simulink model "state_machine_with_obstacle"  (R2016a)
settings: Solver=FixedStepDiscrete  StartTime=0.0  StopTime=100  FixedStep=0.01  MaxStep=0.01  RelTol=1e-3
undefined symbols (not defined in the file): track_3
libraries: lflib x13
settings Model: Creator=The MathWorks, Inc.  LastModifiedBy=bures
settings SolverCC: ZeroCrossAlgorithm=Adaptive
settings DataIOCC: LimitDataPoints=on
settings DebuggingCC: AllowSymbolicDim=off
settings ModelReferenceCC: PropagateSignalLabelsOutOfModel=off
settings GRTTargetCC: GeneratePreprocessorConditionals=Use local settings

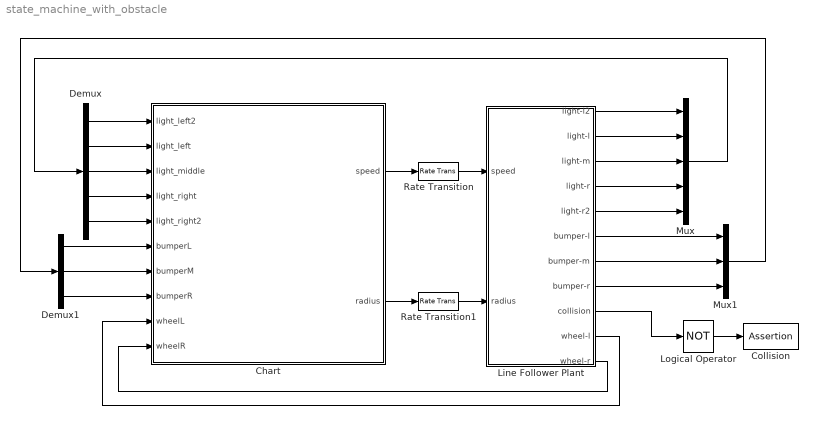
== system state_machine_with_obstacle ==
  Chart : Stateflow chart  TreatAsAtomicUnit=on
  Collision : Assertion
  Demux : Demux  Outputs=5
  Demux1 : Demux  Outputs=3
  Line Follower Plant : Subsystem  mask{initX=506, initY=1050, initAngle=3/2*pi, trackCData=track_3, trackSamplesPerM=1000}
      mask prompts: initX "X (in mm)"; initY "Y (in mm)"; initAngle "Angle (in rad)"; trackCData "Track map"; trackSamplesPerM "Track map samples/m"
  Logical Operator : Logic  Operator=NOT  AllPortsSameDT=off  OutDataTypeStr=boolean
  Mux : Mux  Inputs=5
  Mux1 : Mux  Inputs=3
  Rate Transition : RateTransition  OutPortSampleTime=0.01
  Rate Transition1 : RateTransition  OutPortSampleTime=0.01
  wires:
  Chart/2(radius) -> Rate Transition1/1
  Chart/1(speed) -> Rate Transition/1
  Line Follower Plant/5(light-r2) -> Mux/5
  Line Follower Plant/4(light-r) -> Mux/4
  Line Follower Plant/3(light-m) -> Mux/3
  Line Follower Plant/2(light-l) -> Mux/2
  Line Follower Plant/1(light-l2) -> Mux/1
  Demux/1 -> Chart/1(light_left2)
  Demux/2 -> Chart/2(light_left)
  Demux/3 -> Chart/3(light_middle)
  Demux/4 -> Chart/4(light_right)
  Demux/5 -> Chart/5(light_right2)
  Mux/1 -> Demux/1
  Line Follower Plant/6(bumper-l) -> Mux1/1
  Line Follower Plant/7(bumper-m) -> Mux1/2
  Line Follower Plant/8(bumper-r) -> Mux1/3
  Rate Transition/1 -> Line Follower Plant/1(speed)
  Rate Transition1/1 -> Line Follower Plant/2(radius)
  Demux1/1 -> Chart/6(bumperL)
  Demux1/2 -> Chart/7(bumperM)
  Demux1/3 -> Chart/8(bumperR)
  Mux1/1 -> Demux1/1
  Line Follower Plant/11(wheel-r) -> Chart/10(wheelR)
  Line Follower Plant/10(wheel-l) -> Chart/9(wheelL)
  Line Follower Plant/9(collision) -> Logical Operator/1
  Logical Operator/1 -> Collision/1

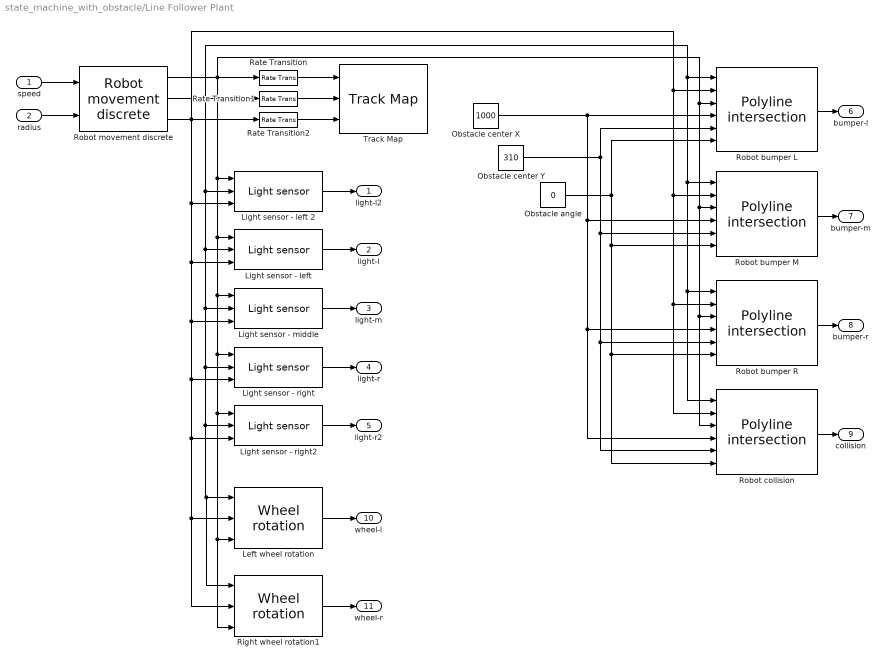
== system state_machine_with_obstacle/Line Follower Plant ==
  speed : Inport
  radius : Inport  Port=2
  Left wheel rotation : lflib/Wheel rotation  wheelPos=[0 140]  initX=initX  initY=initY  initAngle=initAngle
  Light sensor - left : lflib/Light sensor  trackCData=trackCData  trackSamplesPerM=trackSamplesPerM  sensorPos=[150 30]
  Light sensor - left 2 : lflib/Light sensor  trackCData=trackCData  trackSamplesPerM=trackSamplesPerM  sensorPos=[150 70]
  Light sensor - middle : lflib/Light sensor  trackCData=trackCData  trackSamplesPerM=trackSamplesPerM  sensorPos=[150 0]
  Light sensor - right : lflib/Light sensor  trackCData=trackCData  trackSamplesPerM=trackSamplesPerM  sensorPos=[150 -30]
  Light sensor - right2 : lflib/Light sensor  trackCData=trackCData  trackSamplesPerM=trackSamplesPerM  sensorPos=[150 -70]
  Obstacle angle : Constant  Value=0
  Obstacle center X : Constant  Value=1000
  Obstacle center Y : Constant  Value=310
  Rate Transition : RateTransition
  Rate Transition1 : RateTransition
  Rate Transition2 : RateTransition
  Right wheel rotation1 : lflib/Wheel rotation  wheelPos=[0 -140]  initX=initX  initY=initY  initAngle=initAngle
  Robot bumper L : lflib/Polyline intersection  line1=contour_bumperL  line2=contour_obstacle
  Robot bumper M : lflib/Polyline intersection  line1=contour_bumperM  line2=contour_obstacle
  Robot bumper R : lflib/Polyline intersection  line1=contour_bumperR  line2=contour_obstacle
  Robot collision : lflib/Polyline intersection  line1=contour_robot  line2=contour_obstacle
  Robot movement discrete : lflib/Robot movement discrete  initX=initX  initY=initY  initAngle=initAngle
  Track Map : lflib/Track Map  trackCData=trackCData  trackSamplesPerM=trackSamplesPerM
  light-l2 : Outport
  light-l : Outport  Port=2
  light-m : Outport  Port=3
  light-r : Outport  Port=4
  light-r2 : Outport  Port=5
  bumper-l : Outport  Port=6
  bumper-m : Outport  Port=7
  bumper-r : Outport  Port=8
  collision : Outport  Port=9
  wheel-l : Outport  Port=10
  wheel-r : Outport  Port=11
  wires:
  Light sensor - right2/1 -> light-r2/1
  Light sensor - left/1 -> light-l/1
  Light sensor - middle/1 -> light-m/1
  Light sensor - left 2/1 -> light-l2/1
  Light sensor - right/1 -> light-r/1
  radius/1 -> Robot movement discrete/2
  speed/1 -> Robot movement discrete/1
  Robot movement discrete/1 -> Right wheel rotation1/3, Left wheel rotation/3, Light sensor - right2/1, Light sensor - right/1, Light sensor - middle/1, Light sensor - left/1, Light sensor - left 2/1, Robot bumper L/3, Robot bumper M/3, Robot collision/3, Robot bumper R/3, Rate Transition/1
  Robot movement discrete/2 -> Rate Transition1/1, Light sensor - left 2/2, Right wheel rotation1/1, Left wheel rotation/1, Light sensor - right2/2, Light sensor - right/2, Light sensor - middle/2, Light sensor - left/2, Robot bumper L/1, Robot bumper M/1, Robot collision/1, Robot bumper R/1
  Robot movement discrete/3 -> Right wheel rotation1/2, Left wheel rotation/2, Light sensor - right2/3, Light sensor - right/3, Light sensor - middle/3, Light sensor - left/3, Light sensor - left 2/3, Robot bumper L/2, Robot bumper M/2, Robot collision/2, Robot bumper R/2, Rate Transition2/1
  Obstacle center X/1 -> Robot bumper L/4, Robot bumper M/4, Robot collision/4, Robot bumper R/4
  Obstacle center Y/1 -> Robot bumper L/5, Robot bumper M/5, Robot collision/5, Robot bumper R/5
  Obstacle angle/1 -> Robot bumper L/6, Robot bumper M/6, Robot collision/6, Robot bumper R/6
  Robot bumper L/1 -> bumper-l/1
  Robot bumper M/1 -> bumper-m/1
  Robot bumper R/1 -> bumper-r/1
  Robot collision/1 -> collision/1
  Rate Transition/1 -> Track Map/1
  Rate Transition1/1 -> Track Map/2
  Rate Transition2/1 -> Track Map/3
  Right wheel rotation1/1 -> wheel-r/1
  Left wheel rotation/1 -> wheel-l/1

== stateflow chart state_machine_with_obstacle/Chart ==
  state Lap_state [parallel]
    settings: executionOrder=1
    state Init
    state Looking_for_start
    state Start_found
    state Started
    state Beyond_start_line
    (default) -> Init
    Init -> Looking_for_start : /{send(start)}
    Looking_for_start -> Start_found : [light_left2 < 0.5]/{send(stop)}
    Start_found -> Started : after(1,sec)/{send(start)}
    Started -> Beyond_start_line : [light_left2 > 0.5]
  state Driving_state [parallel]
    settings: executionOrder=2
    state Driving
      state Straight
        du:
        speed=100;
        radius=0;
      state Right
        du:
        speed=100;
        radius=100;
      state Left
        du:
        speed=100;
        radius=-100;
      (default) -> Straight
      Straight -> Right [order 1] : [light_middle < 0.5]
      Right -> Straight : [light_middle > 0.5]
      Left -> Straight : [light_right > 0.5]
      Straight -> Left [order 2] : [light_right < 0.5]
    state Still
      du:
      speed=0;
      radius=0;
    Driving -> Still [order 2] : [bumperL || bumperM || bumperR]
    Driving -> Still [order 1] : stop
    Still -> Driving : start
    (default) -> Still
  data: light_left2 input double; light_left input double; light_middle input double; light_right input double; light_right2 input double; speed output double; radius output double; bumperL input boolean; bumperM input boolean; bumperR input boolean; wheelL input; wheelR input
  events: start local FUNCTION_CALL_EVENT; stop local FUNCTION_CALL_EVENT
